simulink model "innerLoop"  (R2024b)
settings: Solver=FixedStepDiscrete  StartTime=0.0  StopTime=0  FixedStep=0.01  RelTol=1e-3
PreLoadFcn:
  | addpath(fileparts(get_param(bdroot,'FileName')));
model workspace (MAT data in the model file):
  H_ship_body = [nan; nan; nan]
  T_body_camera = [nan  nan  nan  nan; nan  nan  nan  nan; nan  nan  nan  nan; nan  nan  nan  nan]
  gear_body = [nan; nan; nan]
settings Model: Creator=yuanjiayi  LastModifiedBy=yuanjiayi

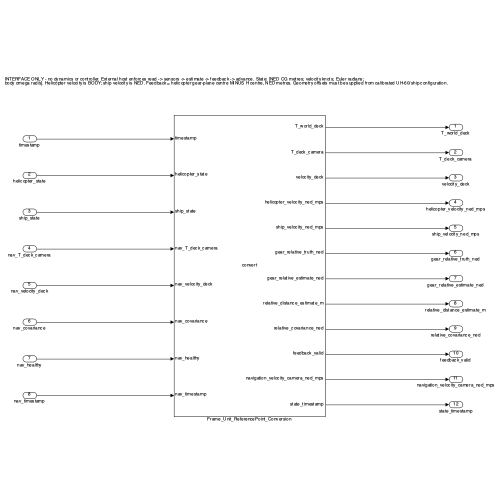
[thumbnail: Simulink's stored preview of the top-level diagram]
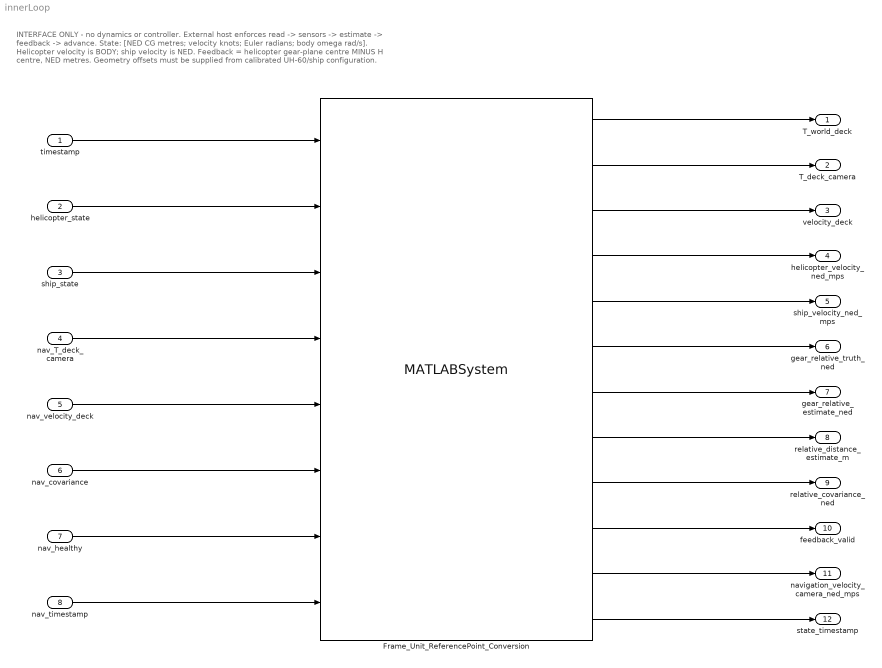
== system innerLoop ==
  note: INTERFACE ONLY - no dynamics or controller. External host enforces read -> sensors -> estimate -> feedback -> advance. State: [NED CG metres; velocity knots; Euler radians;
      | body omega rad/s]. Helicopter velocity is BODY; ship velocity is NED. Feedback = helicopter gear-plane centre MINUS H centre, NED metres. Geometry offsets must be supplied from calibrated UH-60/ship configuration.
  timestamp : Inport  OutDataTypeStr=double  PortDimensions=1
  helicopter_state : Inport  Port=2  OutDataTypeStr=double  PortDimensions=12
  ship_state : Inport  Port=3  OutDataTypeStr=double  PortDimensions=12
  nav_T_deck_camera : Inport  Port=4  OutDataTypeStr=double  PortDimensions=[4 4]
  nav_velocity_deck : Inport  Port=5  OutDataTypeStr=double  PortDimensions=3
  nav_covariance : Inport  Port=6  OutDataTypeStr=double  PortDimensions=[6 6]
  nav_healthy : Inport  Port=7  OutDataTypeStr=double  PortDimensions=1
  nav_timestamp : Inport  Port=8  OutDataTypeStr=double  PortDimensions=1
  Frame_Unit_ReferencePoint_Conversion : MATLABSystem  System=convert  T_body_camera=T_body_camera  H_ship_body=H_ship_body  gear_body=gear_body  SimulateUsing=Interpreted execution
      mask Type: convert
      mask Display:
      | disp('convert');
      | port_label('input',1,'timestamp');
      | port_label('input',2,'helicopter_state');
      | port_label('input',3,'ship_state');
      | port_label('input',4,'nav_T_deck_camera');
      | port_label('input',5,'nav_velocity_deck');
      | port_label('input',6,'nav_covariance');
      | port_label('input',7,'nav_healthy');
      | port_label('input',8,'nav_timestamp');
      | port_label('output',1,'T_world_deck');
      | port_label('output',2,'T_deck_camera');
      | port_label('output',3,'velocity_deck');
      | port_label('output',4,'helicopter_velocity_ned_mps');
      | port_label('output',5,'ship_velocity_ned_mps');
      | port_label('output',6,'gear_relative_truth_ned');
      | port_label('output',7,'gear_relative_estimate_ned');
      | port_label('output',8,'relative_distance_estimate_m');
      | port_label('output',9,'relative_covariance_ned');
      | port_label('output',10,'feedback_valid');
      | port_label('output',11,'navigation_velocity_camera_ned_mps');
      | port_label('output',12,'state_timestamp');
  T_world_deck : Outport
  T_deck_camera : Outport  Port=2
  velocity_deck : Outport  Port=3
  helicopter_velocity_ned_mps : Outport  Port=4
  ship_velocity_ned_mps : Outport  Port=5
  gear_relative_truth_ned : Outport  Port=6
  gear_relative_estimate_ned : Outport  Port=7
  relative_distance_estimate_m : Outport  Port=8
  relative_covariance_ned : Outport  Port=9
  feedback_valid : Outport  Port=10
  navigation_velocity_camera_ned_mps : Outport  Port=11
  state_timestamp : Outport  Port=12
  wires:
  timestamp/1 -> Frame_Unit_ReferencePoint_Conversion/1
  helicopter_state/1 -> Frame_Unit_ReferencePoint_Conversion/2
  ship_state/1 -> Frame_Unit_ReferencePoint_Conversion/3
  nav_T_deck_camera/1 -> Frame_Unit_ReferencePoint_Conversion/4
  nav_velocity_deck/1 -> Frame_Unit_ReferencePoint_Conversion/5
  nav_covariance/1 -> Frame_Unit_ReferencePoint_Conversion/6
  nav_healthy/1 -> Frame_Unit_ReferencePoint_Conversion/7
  nav_timestamp/1 -> Frame_Unit_ReferencePoint_Conversion/8
  Frame_Unit_ReferencePoint_Conversion/1 -> T_world_deck/1
  Frame_Unit_ReferencePoint_Conversion/2 -> T_deck_camera/1
  Frame_Unit_ReferencePoint_Conversion/3 -> velocity_deck/1
  Frame_Unit_ReferencePoint_Conversion/4 -> helicopter_velocity_ned_mps/1
  Frame_Unit_ReferencePoint_Conversion/5 -> ship_velocity_ned_mps/1
  Frame_Unit_ReferencePoint_Conversion/6 -> gear_relative_truth_ned/1
  Frame_Unit_ReferencePoint_Conversion/7 -> gear_relative_estimate_ned/1
  Frame_Unit_ReferencePoint_Conversion/8 -> relative_distance_estimate_m/1
  Frame_Unit_ReferencePoint_Conversion/9 -> relative_covariance_ned/1
  Frame_Unit_ReferencePoint_Conversion/10 -> feedback_valid/1
  Frame_Unit_ReferencePoint_Conversion/11 -> navigation_velocity_camera_ned_mps/1
  Frame_Unit_ReferencePoint_Conversion/12 -> state_timestamp/1
